simulink subsystem "Dynamics"  (R2021a)
settings: Solver=VariableStepAuto  StartTime=0.0  StopTime=10.0  RelTol=1e-3
undefined symbols (not defined in the file): Isc, mu, v0, w0
libraries: sharedutil x1, aerolibutil x1
settings Model: Creator=Laura  LastModifiedBy=Laura

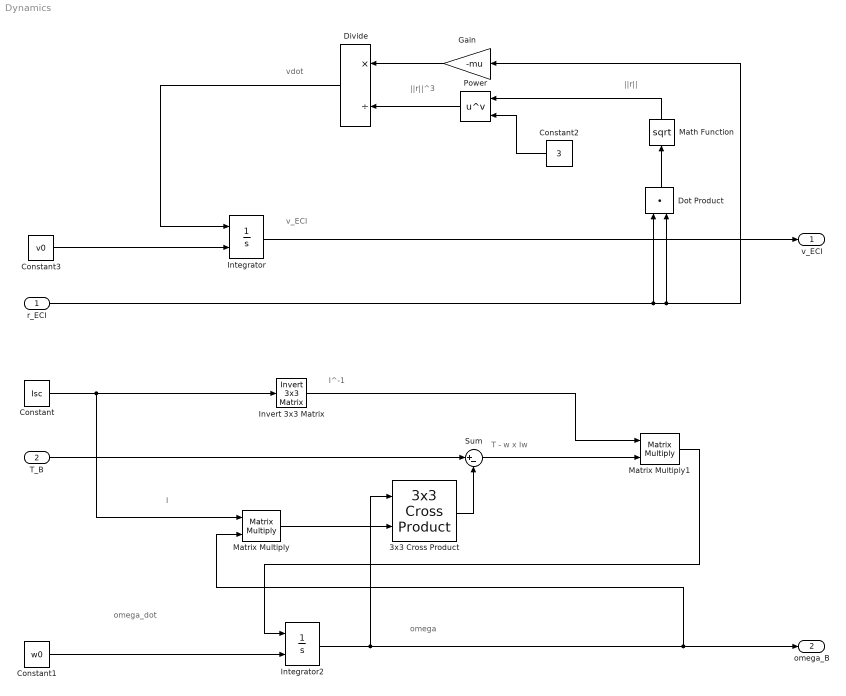
== system Dynamics ==
  note: omega
  note: ||r||
  note: ||r||^3
  note: vdot
  note: omega_dot
  note: T - w x Iw
  note: I^-1
  note: I
  note: v_ECI
  r_ECI : Inport
  T_B : Inport  Port=2
  3x3 Cross Product : sharedutil/3x3 Cross Product  aMode=aMode
      settings: SourceProductBaseCode=AE,PW,DR,MT,UV,VE
  Constant : Constant  Value=Isc
  Constant1 : Constant  Value=w0
  Constant2 : Constant  Value=3
  Constant3 : Constant  Value=v0
  Divide : Product  Inputs=*/
  Dot Product : DotProduct  InputSameDT=on  OutDataTypeStr=Inherit: Inherit via internal rule
  Gain : Gain  Gain=-mu
  Integrator : Integrator  InitialConditionSource=external
  Integrator2 : Integrator  InitialConditionSource=external
  Invert 3x3 Matrix : aerolibutil/Invert  3x3 Matrix
  Math Function : Math  Operator=sqrt  SignedPower=on  SaturateOnIntegerOverflow=on
  Matrix Multiply : Product  Multiplication=Matrix(*)
  Matrix Multiply1 : Product  Multiplication=Matrix(*)
  Power : Math  Operator=pow  SaturateOnIntegerOverflow=on
  Sum : Sum  Inputs=|+-
  v_ECI : Outport
  omega_B : Outport  Port=2
  wires:
  Divide/1 -> Integrator/1
  Integrator2/1 -> omega_B/1, Matrix Multiply/2, 3x3 Cross Product/1
  Sum/1 -> Matrix Multiply1/2
  T_B/1 -> Sum/1
  Invert 3x3 Matrix/1 -> Matrix Multiply1/1
  Math Function/1 -> Power/1
  Gain/1 -> Divide/1
  Power/1 -> Divide/2
  Constant1/1 -> Integrator2/2
  Integrator/1 -> v_ECI/1
  Constant2/1 -> Power/2
  Matrix Multiply1/1 -> Integrator2/1
  Constant3/1 -> Integrator/2
  Matrix Multiply/1 -> 3x3 Cross Product/2
  Constant/1 -> Invert 3x3 Matrix/1, Matrix Multiply/1
  r_ECI/1 -> Dot Product/1, Dot Product/2, Gain/1
  Dot Product/1 -> Math Function/1
  3x3 Cross Product/1 -> Sum/2
